simulink library "LargeScaleSimLib_old"  (R2019a)
settings: Solver=VariableStepAuto  StartTime=0.0  StopTime=10.0  RelTol=1e-3
undefined symbols (not defined in the file or in its folder): Objects
libraries: genericAgentLib x2
settings Model: Creator=akshay  LastModifiedBy=akshay

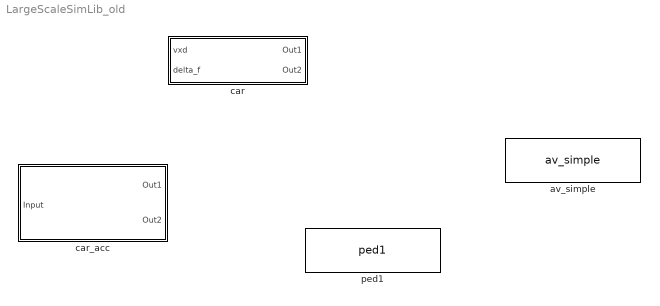
== system LargeScaleSimLib_old ==
  av_simple : genericAgentLib/av_simple  obj=Objects{6}
  car : Subsystem  AncestorBlock=genericAgentLib/car  mask{obj=Objects{1}}
      mask prompts: obj "object"
      mask init:
      | set_param([gcb,'/ToWS'],'VariableName',obj.NameStrh)
  car_acc : Subsystem  mask{obj=Objects{1}}
      mask prompts: obj "object"
  ped1 : genericAgentLib/ped1  obj=Objects{3}

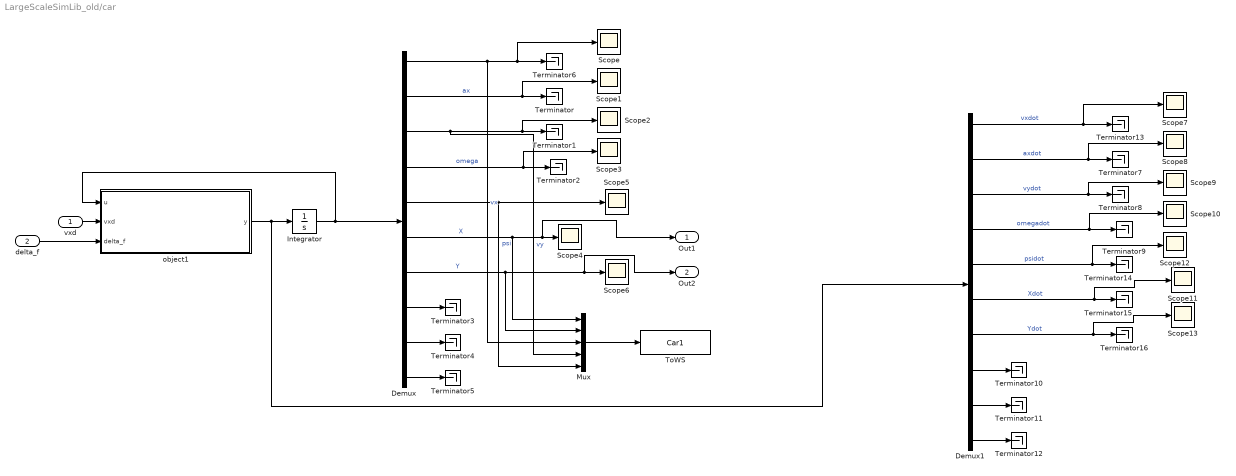
== system LargeScaleSimLib_old/car ==
  "vxd " : Inport
  delta_f : Inport  Port=2
  Demux : Demux  Outputs=10
  Demux1 : Demux  Outputs=10
  Integrator : Integrator  InitialCondition=obj.init
  Mux : Mux  Inputs=5
  Scope{,1..13} (14 alike) : Scope
  Terminator{,1..16} (17 alike) : Terminator
  ToWS : ToWorkspace  VariableName=Car1  SaveFormat=Timeseries  SampleTime=-1
  object1 : MATLAB Function  TreatAsAtomicUnit=on
  Out1 : Outport
  Out2 : Outport  Port=2
  wires:
  Integrator/1 -> Demux/1, object1/1(u)
  delta_f/1 -> object1/3(delta_f)
  Demux/1 -> Mux/3, Scope/1, Terminator6/1  "vx"
  Demux/2 -> Scope1/1, Terminator/1  "ax"
  Demux/3 -> Mux/4, Scope2/1, Terminator1/1  "vy"
  Demux/4 -> Scope3/1, Terminator2/1  "omega"
  Demux/5 -> Mux/5, Scope5/1  "psi"
  Demux/6 -> Mux/1, Out1/1, Scope4/1  "X"
  Demux/7 -> Mux/2, Out2/1, Scope6/1  "Y"
  Demux/8 -> Terminator3/1
  Demux/9 -> Terminator4/1
  Demux/10 -> Terminator5/1
  Demux1/10 -> Terminator12/1
  Demux1/9 -> Terminator11/1
  Demux1/8 -> Terminator10/1
  Demux1/7 -> Terminator16/1, Scope13/1  "Ydot"
  Demux1/6 -> Terminator15/1, Scope11/1  "Xdot"
  Demux1/5 -> Terminator14/1, Scope12/1  "psidot"
  Demux1/4 -> Terminator9/1, Scope10/1  "omegadot"
  Demux1/3 -> Terminator8/1, Scope9/1  "vydot"
  Demux1/2 -> Terminator7/1, Scope8/1  "axdot"
  Demux1/1 -> Terminator13/1, Scope7/1  "vxdot"
  object1/1(y) -> Demux1/1, Integrator/1
  Mux/1 -> ToWS/1
  "vxd "/1 -> object1/2(vxd)

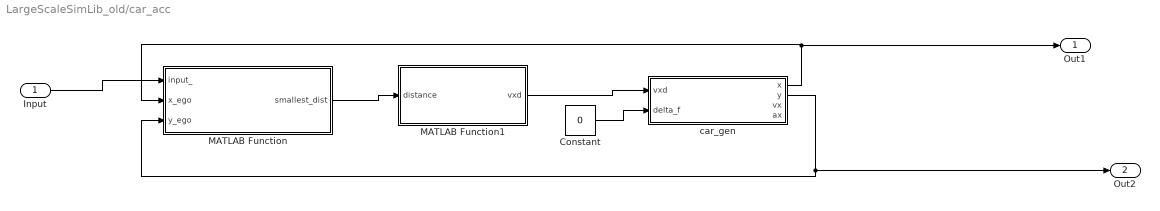
== system LargeScaleSimLib_old/car_acc ==
  Input : Inport
  Constant : Constant  Value=0
  MATLAB Function : MATLAB Function  TreatAsAtomicUnit=on
  MATLAB Function1 : MATLAB Function  TreatAsAtomicUnit=on
  car_gen : Subsystem  AncestorBlock=genericAgentLib/car  mask{obj=obj}
      mask prompts: obj "object"
      mask init:
      | set_param([gcb,'/ToWS'],'VariableName',obj.NameStrh)
  Out1 : Outport
  Out2 : Outport  Port=2
  wires:
  car_gen/1(x) -> Out1/1, MATLAB Function/2(x_ego)
  car_gen/2(y) -> Out2/1, MATLAB Function/3(y_ego)
  Input/1 -> MATLAB Function/1(input_)
  MATLAB Function/1(smallest_dist) -> MATLAB Function1/1(distance)
  Constant/1 -> car_gen/2(delta_f)
  MATLAB Function1/1(vxd) -> car_gen/1("vxd ")

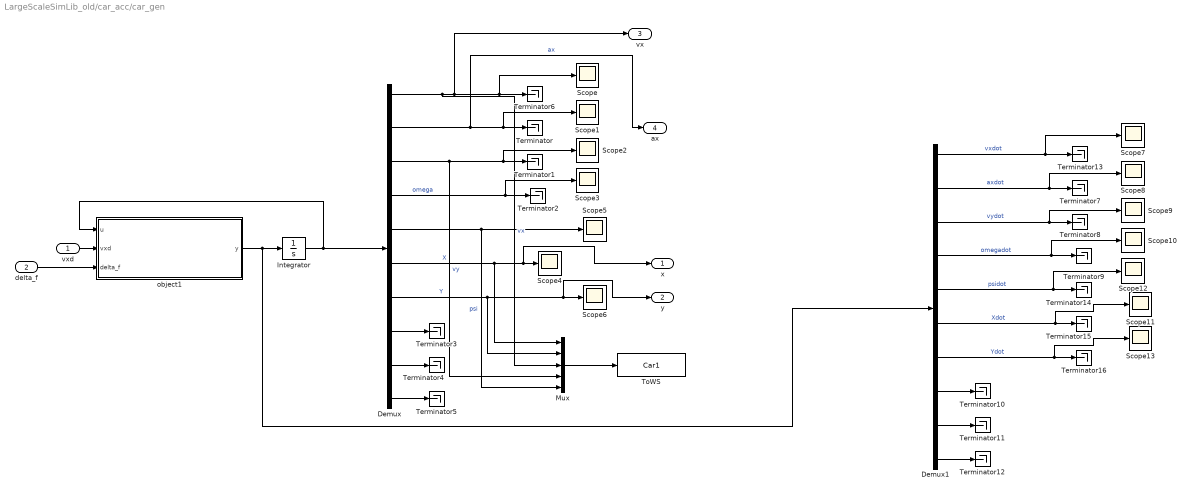
== system LargeScaleSimLib_old/car_acc/car_gen ==
  "vxd " : Inport
  delta_f : Inport  Port=2
  Demux : Demux  Outputs=10
  Demux1 : Demux  Outputs=10
  Integrator : Integrator  InitialCondition=obj.init
  Mux : Mux  Inputs=5
  Scope{,1..13} (14 alike) : Scope
  Terminator{,1..16} (17 alike) : Terminator
  ToWS : ToWorkspace  VariableName=Car1  SaveFormat=Timeseries  SampleTime=-1
  object1 : MATLAB Function  TreatAsAtomicUnit=on
  x : Outport
  y : Outport  Port=2
  vx : Outport  Port=3
  "ax " : Outport  Port=4
  wires:
  Integrator/1 -> Demux/1, object1/1(u)
  delta_f/1 -> object1/3(delta_f)
  Demux/1 -> Mux/3, vx/1, Scope/1, Terminator6/1  "vx"
  Demux/2 -> "ax "/1, Scope1/1, Terminator/1  "ax"
  Demux/3 -> Mux/4, Scope2/1, Terminator1/1  "vy"
  Demux/4 -> Scope3/1, Terminator2/1  "omega"
  Demux/5 -> Mux/5, Scope5/1  "psi"
  Demux/6 -> Mux/1, x/1, Scope4/1  "X"
  Demux/7 -> Mux/2, y/1, Scope6/1  "Y"
  Demux/8 -> Terminator3/1
  Demux/9 -> Terminator4/1
  Demux/10 -> Terminator5/1
  Demux1/10 -> Terminator12/1
  Demux1/9 -> Terminator11/1
  Demux1/8 -> Terminator10/1
  Demux1/7 -> Terminator16/1, Scope13/1  "Ydot"
  Demux1/6 -> Terminator15/1, Scope11/1  "Xdot"
  Demux1/5 -> Terminator14/1, Scope12/1  "psidot"
  Demux1/4 -> Terminator9/1, Scope10/1  "omegadot"
  Demux1/3 -> Terminator8/1, Scope9/1  "vydot"
  Demux1/2 -> Terminator7/1, Scope8/1  "axdot"
  Demux1/1 -> Terminator13/1, Scope7/1  "vxdot"
  object1/1(y) -> Demux1/1, Integrator/1
  Mux/1 -> ToWS/1
  "vxd "/1 -> object1/2(vxd)

== matlab function LargeScaleSimLib_old/car_acc/car_gen/object1 ==
  data: u input size=10; vxd input size=1; delta_f input size=1; y output size=10; obj parameter
function y = fcn(u,vxd, delta_f, obj)

vx = u(1);
ax = u(2);
vy = u(3);
omega = u(4);
psi = u(5);
X = u(6);
Y = u(7);

if abs(vx)> obj.vx_threshold1
    alpha_f = delta_f * pi/180 - (vy + omega * obj.lf) / vx;
    alpha_r = - (vy - omega * obj.lr) / vx;
else
    alpha_f = 0;
    alpha_r = 0;
end

Fx = obj.m * ax;
Fyf = min(obj.Fyfmax,obj.Calpha_f * alpha_f);
Fyr = min(obj.Fyrmax, obj.Calpha_r * alpha_r);
Fy = Fyf + Fyr;

M  = Fyf * obj.lf - Fyr * obj.lr;

omegadot = M / obj.I;
%        vxdot = Fx / obj.m + omega * vy;
vxdot = ax;
axdot = - 2 * obj.longctl.psi * obj.longctl.w* ax - (obj.longctl.w)^2 * (vx - vxd);
vydot = Fy / obj.m - omega * vx;
psidot = omega;
t1 = TF(psi) * [vx;vy];
Xdot = t1(1);
Ydot = t1(2);
y = [vxdot, axdot, vydot, omegadot, psidot, Xdot, Ydot, 0 0 0]';
end

function y = TF(psi)
y = [cos(psi), sin(psi); -sin(psi), cos(psi)];
end

== matlab function LargeScaleSimLib_old/car/object1 ==
  data: u input size=10; vxd input size=1; delta_f input size=1; y output size=10; obj parameter
function y = fcn(u,vxd, delta_f, obj)

vx = u(1);
ax = u(2);
vy = u(3);
omega = u(4);
psi = u(5);
X = u(6);
Y = u(7);

if abs(vx)> obj.vx_threshold1
    alpha_f = delta_f * pi/180 - (vy + omega * obj.lf) / vx;
    alpha_r = - (vy - omega * obj.lr) / vx;
else
    alpha_f = 0;
    alpha_r = 0;
end

Fx = obj.m * ax;
Fyf = min(obj.Fyfmax,obj.Calpha_f * alpha_f);
Fyr = min(obj.Fyrmax, obj.Calpha_r * alpha_r);
Fy = Fyf + Fyr;

M  = Fyf * obj.lf - Fyr * obj.lr;

omegadot = M / obj.I;
%        vxdot = Fx / obj.m + omega * vy;
vxdot = ax;
axdot = - 2 * obj.longctl.psi * obj.longctl.w* ax - (obj.longctl.w)^2 * (vx - vxd);
vydot = Fy / obj.m - omega * vx;
psidot = omega;
t1 = TF(psi) * [vx;vy];
Xdot = t1(1);
Ydot = t1(2);
y = [vxdot, axdot, vydot, omegadot, psidot, Xdot, Ydot, 0 0 0]';
end

function y = TF(psi)
y = [cos(psi), sin(psi); -sin(psi), cos(psi)];
end

== matlab function LargeScaleSimLib_old/car_acc/MATLAB Function ==
  data: input_ input; smallest_dist output; x_ego input; y_ego input
function smallest_dist = sensor(input_, x_ego, y_ego)

smallest_d = inf;
x = 1;


for c = 1:(length(input_)/2)

    temp_d = sqrt((x_ego - input_(x))^2+(y_ego-input_(x+1))^2);
    
    if ((smallest_d > temp_d) && (temp_d > 1) &&((input_(x) > x_ego)))% &&~(y_ego == input_(x+1)) )
        
        smallest_d = temp_d;
        
    end
    x = x+2;
    
end


smallest_dist = smallest_d;

== matlab function LargeScaleSimLib_old/car_acc/MATLAB Function1 ==
  data: vxd output; distance input
function vxd = fcn(distance)

d_thres1 = 80;
d_thres2 = 100;
vx_ref = 30;
kp = 0.001;
cc = 1;
vxd = 1;
if(cc)
    v_des = vx_ref;
    if(distance <= d_thres1)
        cc = 0;
    else
        cc = 1;%redunadnt statement
    end
else 
    v_des = vx_ref - kp*(d_thres1 - distance);
    if(distance > d_thres2)
        cc = 1;
    else
        cc = 0;%redundant statement
    end
end

% 
% if((distance <=  d_thres1))
%     v_des = vx_ref - kp*(d_thres1 - distance);
% elseif (distance > d_thres2)
%     v_des = vx_ref;
% else
%     v_des = vx_ref;
% end


vxd = v_des;
